simulink model "myTwoInOne3D"  (R2024a)
settings: Solver=VariableStepAuto  StartTime=0.0  StopTime=10.0  RelTol=1e-3
InitFcn:
  | close all;
  | clear all;
  | % 入力格子（行列）作成
  | [x1, x2] = meshgrid(-1:0.2:0.8, -1:0.2:0.8);
  | y = zeros(10, 10);
StopFcn:
  | y = out.y.Data;
  | surf(x1, x2, y);
  | colorbar;
undefined symbols (not defined in the file or in its folder): x1, x2
libraries: neural x1
settings Model: Creator=mashi  LastModifiedBy=mashi

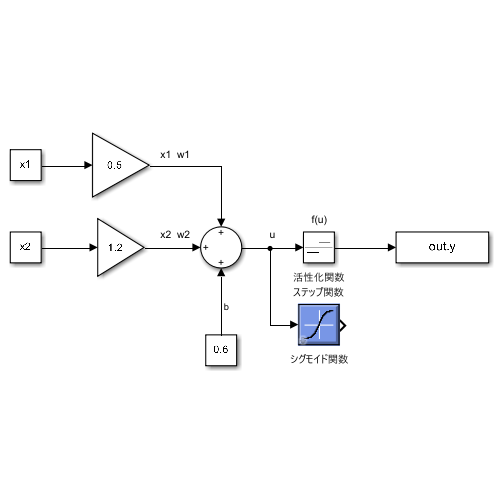
[thumbnail: Simulink's stored preview of the top-level diagram]
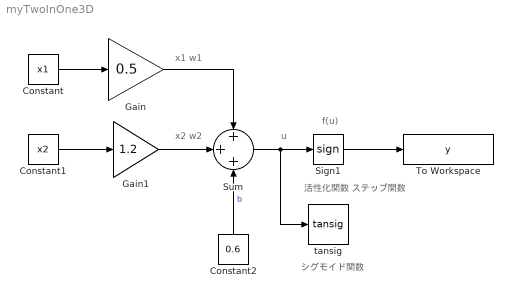
== system myTwoInOne3D ==
  note: シグモイド関数
  note: 活性化関数
      | ステップ関数
  note: f(u)
  note: x1 w1
  note: u
  note: x2 w2
  Constant : Constant  Value=x1
  Constant1 : Constant  Value=x2
  Constant2 : Constant  Value=0.6
  Gain : Gain  Gain=0.5
  Gain1 : Gain  Gain=1.2
  Sign1 : Signum
  Sum : Sum  Inputs=+++
  To Workspace : ToWorkspace  VariableName=y  SaveFormat=Timeseries  SampleTime=-1
  tansig : neural/Transfer Functions/tansig
  wires:
  Constant/1 -> Gain/1
  Constant1/1 -> Gain1/1
  Gain/1 -> Sum/1
  Gain1/1 -> Sum/2
  Constant2/1 -> Sum/3  "b"
  Sum/1 -> Sign1/1, tansig/1
  Sign1/1 -> To Workspace/1
